simulink model "green_joint_mit_mode_1615_harness"  (R2023b)
settings: Solver=FixedStepDiscrete  StartTime=0.0  StopTime=GJDT_MIT_StopTime_s  FixedStep=GJDT_Ts  RelTol=1e-3
values from neighbouring files (symbols this model uses):
  GJDT_MIT_BOutput_NmSPerRad = single(      motor.output_viscous_damping_nm_s_per_rad)    [setup_green_joint_mit_mode_1615_harness.m]
  GJDT_MIT_CurrentAlpha = single(1.0 - exp(-GJDT_Ts /      GJDT_MIT_CurrentTau_s))    [setup_green_joint_mit_mode_1615_harness.m]
  GJDT_MIT_FfTorque_Nm = single(0.0)    [setup_green_joint_mit_mode_1615_harness.m]
  GJDT_MIT_FrictionSmoothing_RadS = single(0.02)    [setup_green_joint_mit_mode_1615_harness.m]
  GJDT_MIT_IqLimit_A = single(GJDT_ModuleConfig.defaults.torque_limit_a)    [setup_green_joint_mit_mode_1615_harness.m]
  GJDT_MIT_JOutput_KgM2 = single(motor.output_equivalent_inertia_kg_m2)    [setup_green_joint_mit_mode_1615_harness.m]
  GJDT_MIT_Kd_APerRadS = single(kd_nm_s_per_rad / kt_output)    [setup_green_joint_mit_mode_1615_harness.m]
  GJDT_MIT_Kp_APerRad = single(kp_nm_per_rad / kt_output)    [setup_green_joint_mit_mode_1615_harness.m]
  GJDT_MIT_KtOutput_NmPerA = single(motor.torque_constant * motor.gear_ratio)    [setup_green_joint_mit_mode_1615_harness.m]
  GJDT_MIT_PosStepTime_s = 0.020    (= 0.02)    [setup_green_joint_mit_mode_1615_harness.m]
  GJDT_MIT_PosTarget_Rad = single(0.20)    [setup_green_joint_mit_mode_1615_harness.m]
  GJDT_MIT_TbiasOutput_Nm = single(motor.output_torque_bias_nm)    [setup_green_joint_mit_mode_1615_harness.m]
  GJDT_MIT_TcOutput_Nm = single(motor.output_coulomb_friction_nm)    [setup_green_joint_mit_mode_1615_harness.m]
  GJDT_MIT_TorqueToIq_APerNm = single(1.0 /      double(GJDT_MIT_KtOutput_NmPerA))    [setup_green_joint_mit_mode_1615_harness.m]
  GJDT_MIT_VelTarget_RadS = single(0.0)    [setup_green_joint_mit_mode_1615_harness.m]
  GJDT_Ts = 50e-6    (= 5e-05)    [setup_green_joint_current_loop_twin.m]
Description:
  | Visible MIT 1615 harness. TestSupervisor and plant are simulation-only; MIT algorithm is referenced from MBD core.
settings Model: DataDictionary=green_joint_mit_impedance_interface.sldd  Creator=user  LastModifiedBy=user
settings DebuggingCC: ParameterPrecisionLossMsg=none

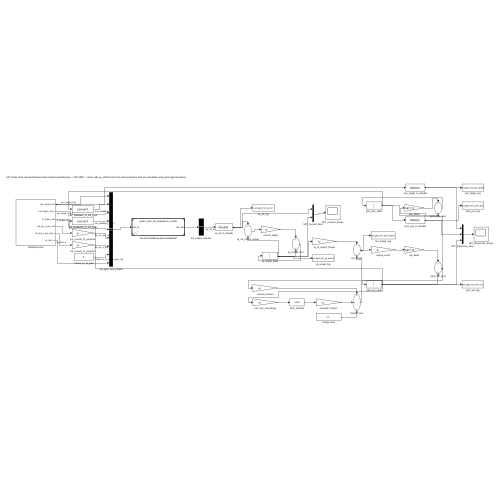
[thumbnail: Simulink's stored preview of the top-level diagram]
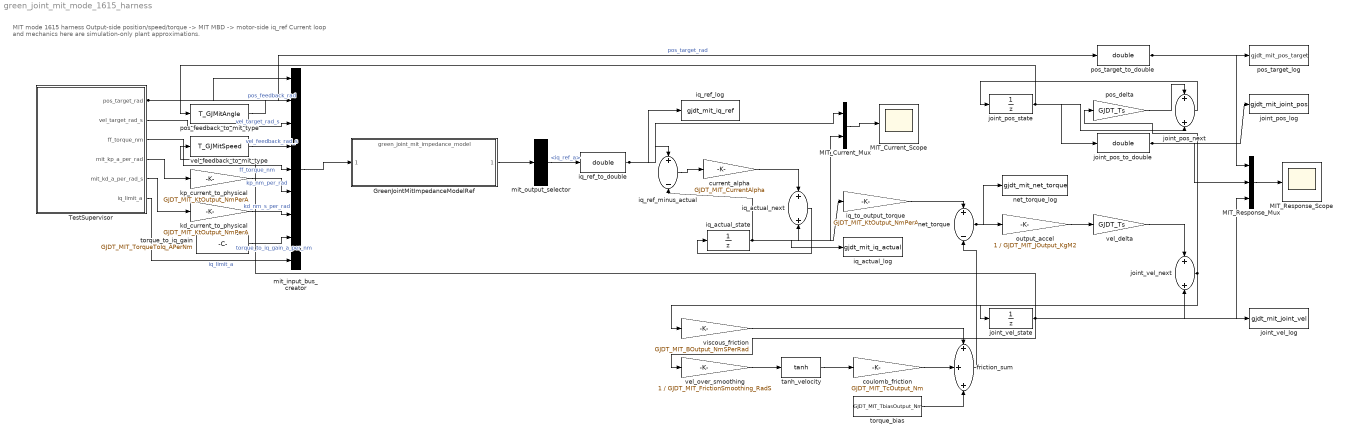
== system green_joint_mit_mode_1615_harness ==
  note: MIT mode 1615 harness\nOutput-side position/speed/torque -> MIT MBD -> motor-side iq_ref\nCurrent loop and mechanics here are simulation-only plant approximations.
  GreenJointMitImpedanceModelRef : ModelReference  ModelNameDialog=green_joint_mit_impedance_model  SimulationMode=Normal  ModelReferenceVersion=1.1
  MIT_Current_Mux : Mux  Inputs=2
  MIT_Current_Scope : Scope
  MIT_Response_Mux : Mux  Inputs=3
  MIT_Response_Scope : Scope
  TestSupervisor : Subsystem
  coulomb_friction : Gain  Gain=GJDT_MIT_TcOutput_Nm
  current_alpha : Gain  Gain=GJDT_MIT_CurrentAlpha
  friction_sum : Sum  Inputs=+++
  iq_actual_log : ToWorkspace  VariableName=gjdt_mit_iq_actual  SaveFormat=Structure With Time  SampleTime=-1
  iq_actual_next : Sum
  iq_actual_state : UnitDelay  SampleTime=GJDT_Ts  HasFrameUpgradeWarning=on
  iq_ref_log : ToWorkspace  VariableName=gjdt_mit_iq_ref  SaveFormat=Structure With Time  SampleTime=-1
  iq_ref_minus_actual : Sum  Inputs=+-
  iq_ref_to_double : DataTypeConversion  OutDataTypeStr=double  SaturateOnIntegerOverflow=off  RndMeth=Floor
  iq_to_output_torque : Gain  Gain=GJDT_MIT_KtOutput_NmPerA
  joint_pos_log : ToWorkspace  VariableName=gjdt_mit_joint_pos  SaveFormat=Structure With Time  SampleTime=-1
  joint_pos_next : Sum
  joint_pos_state : UnitDelay  SampleTime=GJDT_Ts  HasFrameUpgradeWarning=on
  joint_pos_to_double : DataTypeConversion  OutDataTypeStr=double  SaturateOnIntegerOverflow=off  RndMeth=Floor
  joint_vel_log : ToWorkspace  VariableName=gjdt_mit_joint_vel  SaveFormat=Structure With Time  SampleTime=-1
  joint_vel_next : Sum
  joint_vel_state : UnitDelay  SampleTime=GJDT_Ts  HasFrameUpgradeWarning=on
  kd_current_to_physical : Gain  Gain=GJDT_MIT_KtOutput_NmPerA  OutDataTypeStr=T_GJMitGain
  kp_current_to_physical : Gain  Gain=GJDT_MIT_KtOutput_NmPerA  OutDataTypeStr=T_GJMitGain
  mit_input_bus_creator : BusCreator  Inputs=9  OutDataTypeStr=Bus: green_joint_mit_input_t  NonVirtualBus=on
  mit_output_selector : BusSelector  OutputSignals=iq_ref_a
  net_torque : Sum  Inputs=+-
  net_torque_log : ToWorkspace  VariableName=gjdt_mit_net_torque  SaveFormat=Structure With Time  SampleTime=-1
  output_accel : Gain  Gain=1 / GJDT_MIT_JOutput_KgM2
  pos_delta : Gain  Gain=GJDT_Ts
  pos_feedback_to_mit_type : DataTypeConversion  OutDataTypeStr=T_GJMitAngle  SaturateOnIntegerOverflow=off  RndMeth=Floor
  pos_target_log : ToWorkspace  VariableName=gjdt_mit_pos_target  SaveFormat=Structure With Time  SampleTime=-1
  pos_target_to_double : DataTypeConversion  OutDataTypeStr=double  SaturateOnIntegerOverflow=off  RndMeth=Floor
  tanh_velocity : Trigonometry  Operator=tanh
  torque_bias : Constant  Value=GJDT_MIT_TbiasOutput_Nm  SampleTime=GJDT_Ts
  torque_to_iq_gain : Constant  Value=GJDT_MIT_TorqueToIq_APerNm  OutDataTypeStr=T_GJMitGain  SampleTime=GJDT_Ts
  vel_delta : Gain  Gain=GJDT_Ts
  vel_feedback_to_mit_type : DataTypeConversion  OutDataTypeStr=T_GJMitSpeed  SaturateOnIntegerOverflow=off  RndMeth=Floor
  vel_over_smoothing : Gain  Gain=1 / GJDT_MIT_FrictionSmoothing_RadS
  viscous_friction : Gain  Gain=GJDT_MIT_BOutput_NmSPerRad
  wires:
  TestSupervisor/1(pos_target_rad) -> mit_input_bus_creator/1, pos_target_to_double/1  "pos_target_rad"
  TestSupervisor/2(vel_target_rad_s) -> mit_input_bus_creator/3  "vel_target_rad_s"
  TestSupervisor/3(ff_torque_nm) -> mit_input_bus_creator/5  "ff_torque_nm"
  TestSupervisor/4(mit_kp_a_per_rad) -> kp_current_to_physical/1
  TestSupervisor/5(mit_kd_a_per_rad_s) -> kd_current_to_physical/1
  TestSupervisor/6(iq_limit_a) -> mit_input_bus_creator/9  "iq_limit_a"
  joint_pos_state/1 -> pos_feedback_to_mit_type/1, joint_pos_next/2, joint_pos_to_double/1
  joint_vel_state/1 -> vel_feedback_to_mit_type/1, viscous_friction/1, vel_over_smoothing/1, joint_vel_next/2, joint_vel_log/1, MIT_Response_Mux/3
  pos_feedback_to_mit_type/1 -> mit_input_bus_creator/2  "pos_feedback_rad"
  vel_feedback_to_mit_type/1 -> mit_input_bus_creator/4  "vel_feedback_rad_s"
  kp_current_to_physical/1 -> mit_input_bus_creator/6  "kp_nm_per_rad"
  kd_current_to_physical/1 -> mit_input_bus_creator/7  "kd_nm_s_per_rad"
  torque_to_iq_gain/1 -> mit_input_bus_creator/8  "torque_to_iq_gain_a_per_nm"
  mit_input_bus_creator/1 -> GreenJointMitImpedanceModelRef/1
  GreenJointMitImpedanceModelRef/1 -> mit_output_selector/1
  mit_output_selector/1 -> iq_ref_to_double/1  "<iq_ref_a>"
  iq_ref_to_double/1 -> iq_ref_minus_actual/1, iq_ref_log/1, MIT_Current_Mux/1
  iq_actual_state/1 -> iq_ref_minus_actual/2, iq_actual_next/2, iq_to_output_torque/1, iq_actual_log/1, MIT_Current_Mux/2
  iq_ref_minus_actual/1 -> current_alpha/1
  current_alpha/1 -> iq_actual_next/1
  iq_actual_next/1 -> iq_actual_state/1
  iq_to_output_torque/1 -> net_torque/1
  vel_over_smoothing/1 -> tanh_velocity/1
  tanh_velocity/1 -> coulomb_friction/1
  viscous_friction/1 -> friction_sum/1
  coulomb_friction/1 -> friction_sum/2
  torque_bias/1 -> friction_sum/3
  friction_sum/1 -> net_torque/2
  net_torque/1 -> output_accel/1, net_torque_log/1
  output_accel/1 -> vel_delta/1
  vel_delta/1 -> joint_vel_next/1
  joint_vel_next/1 -> joint_vel_state/1, pos_delta/1
  pos_delta/1 -> joint_pos_next/1
  joint_pos_next/1 -> joint_pos_state/1
  pos_target_to_double/1 -> pos_target_log/1, MIT_Response_Mux/1
  joint_pos_to_double/1 -> joint_pos_log/1, MIT_Response_Mux/2
  MIT_Response_Mux/1 -> MIT_Response_Scope/1
  MIT_Current_Mux/1 -> MIT_Current_Scope/1

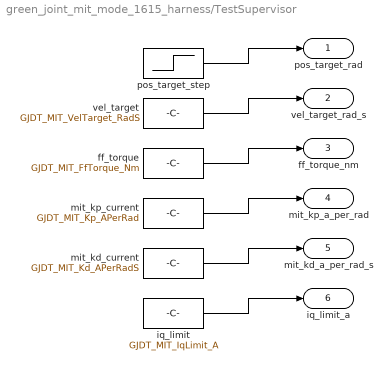
== system green_joint_mit_mode_1615_harness/TestSupervisor ==
  ff_torque : Constant  Value=GJDT_MIT_FfTorque_Nm  OutDataTypeStr=T_GJMitTorque  SampleTime=GJDT_Ts
  iq_limit : Constant  Value=GJDT_MIT_IqLimit_A  OutDataTypeStr=T_GJMitCurrent  SampleTime=GJDT_Ts
  mit_kd_current : Constant  Value=GJDT_MIT_Kd_APerRadS  OutDataTypeStr=T_GJMitGain  SampleTime=GJDT_Ts
  mit_kp_current : Constant  Value=GJDT_MIT_Kp_APerRad  OutDataTypeStr=T_GJMitGain  SampleTime=GJDT_Ts
  pos_target_step : Step  Time=GJDT_MIT_PosStepTime_s  Before=single(0)  After=GJDT_MIT_PosTarget_Rad  OutDataTypeStr=T_GJMitAngle  SampleTime=GJDT_Ts
  vel_target : Constant  Value=GJDT_MIT_VelTarget_RadS  OutDataTypeStr=T_GJMitSpeed  SampleTime=GJDT_Ts
  pos_target_rad : Outport
  vel_target_rad_s : Outport  Port=2
  ff_torque_nm : Outport  Port=3
  mit_kp_a_per_rad : Outport  Port=4
  mit_kd_a_per_rad_s : Outport  Port=5
  iq_limit_a : Outport  Port=6
  wires:
  pos_target_step/1 -> pos_target_rad/1
  vel_target/1 -> vel_target_rad_s/1
  ff_torque/1 -> ff_torque_nm/1
  mit_kp_current/1 -> mit_kp_a_per_rad/1
  mit_kd_current/1 -> mit_kd_a_per_rad_s/1
  iq_limit/1 -> iq_limit_a/1
